simulink subsystem "control_initializer"  (R2023a)
settings: Solver=VariableStepAuto  StartTime=0.0  StopTime=10.0  RelTol=1e-3
libraries: sharedtransform x1
settings Model: Creator=thesa  LastModifiedBy=thesa

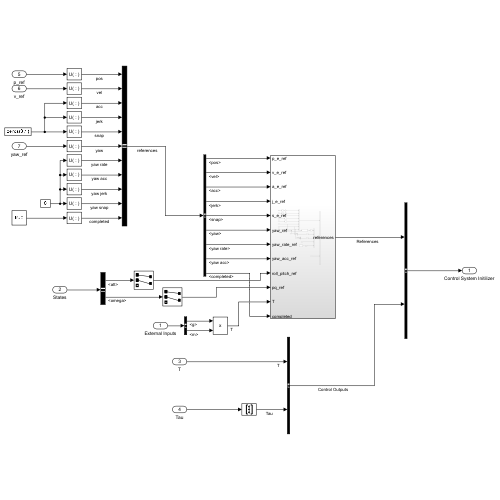
[thumbnail: Simulink's stored preview of the top-level diagram]
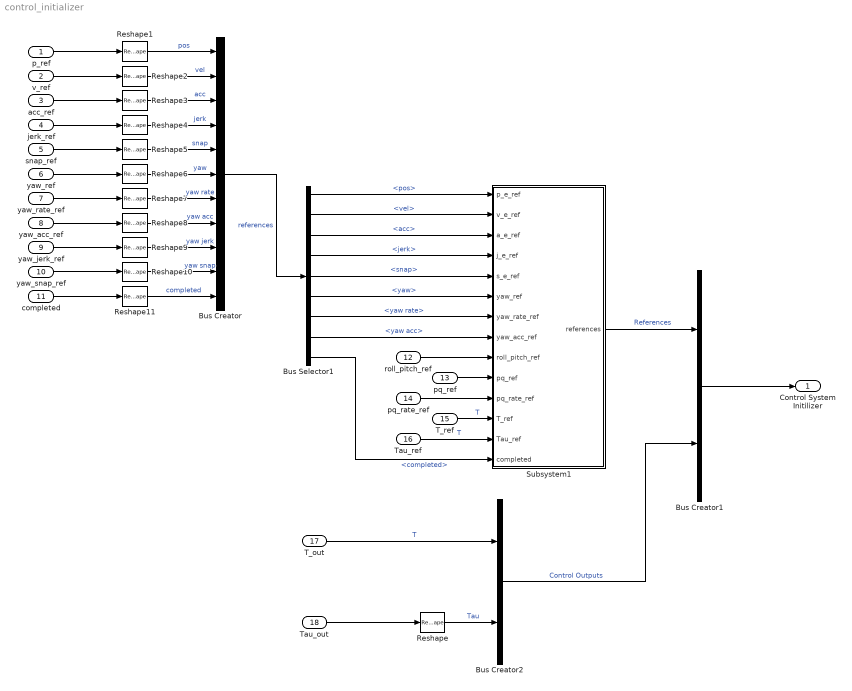
== system control_initializer ==
  p_ref : Inport
  v_ref : Inport  Port=2
  acc_ref : Inport  Port=3
  jerk_ref : Inport  Port=4
  snap_ref : Inport  Port=5
  yaw_ref : Inport  Port=6
  yaw_rate_ref : Inport  Port=7
  yaw_acc_ref : Inport  Port=8
  yaw_jerk_ref : Inport  Port=9
  yaw_snap_ref : Inport  Port=10
  completed : Inport  Port=11
  roll_pitch_ref : Inport  Port=12
  pq_ref : Inport  Port=13
  pq_rate_ref : Inport  Port=14
  T_ref : Inport  Port=15
  Tau_ref : Inport  Port=16
  T_out : Inport  Port=17
  Tau_out : Inport  Port=18
  Bus Creator : BusCreator  Inputs=11
  Bus Creator1 : BusCreator  Inputs=2
  Bus Creator2 : BusCreator  Inputs=2
  Bus Selector1 : BusSelector  OutputSignals=pos,vel,acc,jerk,snap,yaw,yaw rate,yaw acc,completed
  Reshape : Reshape  OutputDimensionality=Column vector (2-D)
  Reshape{1..11} (11 alike) : Reshape
  Subsystem1 : Subsystem
  Control System Initilizer : Outport
  wires:
  Reshape9/1 -> Bus Creator/9  "yaw jerk"
  Reshape5/1 -> Bus Creator/5  "snap"
  Reshape2/1 -> Bus Creator/2  "vel"
  Reshape6/1 -> Bus Creator/6  "yaw"
  T_out/1 -> Bus Creator2/1  "T"
  Bus Selector1/7 -> Subsystem1/7(yaw_rate_ref)  "<yaw rate>"
  Reshape11/1 -> Bus Creator/11  "completed"
  Reshape8/1 -> Bus Creator/8  "yaw acc"
  Reshape10/1 -> Bus Creator/10  "yaw snap"
  Subsystem1/1(references) -> Bus Creator1/1  "References"
  Bus Selector1/2 -> Subsystem1/2(v_e_ref)  "<vel>"
  Bus Selector1/4 -> Subsystem1/4(j_e_ref)  "<jerk>"
  p_ref/1 -> Reshape1/1
  Reshape1/1 -> Bus Creator/1  "pos"
  Bus Selector1/5 -> Subsystem1/5(s_e_ref)  "<snap>"
  Bus Creator1/1 -> Control System Initilizer/1
  Bus Selector1/9 -> Subsystem1/14(completed)  "<completed>"
  Reshape7/1 -> Bus Creator/7  "yaw rate"
  Bus Selector1/6 -> Subsystem1/6(yaw_ref)  "<yaw>"
  Bus Creator/1 -> Bus Selector1/1  "references"
  Bus Creator2/1 -> Bus Creator1/2  "Control Outputs"
  T_ref/1 -> Subsystem1/12(T_ref)  "T"
  Bus Selector1/1 -> Subsystem1/1(p_e_ref)  "<pos>"
  Reshape4/1 -> Bus Creator/4  "jerk"
  v_ref/1 -> Reshape2/1
  Bus Selector1/3 -> Subsystem1/3(a_e_ref)  "<acc>"
  yaw_ref/1 -> Reshape6/1
  Bus Selector1/8 -> Subsystem1/8(yaw_acc_ref)  "<yaw acc>"
  Reshape/1 -> Bus Creator2/2  "Tau"
  Tau_out/1 -> Reshape/1
  Reshape3/1 -> Bus Creator/3  "acc"
  jerk_ref/1 -> Reshape4/1
  acc_ref/1 -> Reshape3/1
  snap_ref/1 -> Reshape5/1
  yaw_rate_ref/1 -> Reshape7/1
  yaw_acc_ref/1 -> Reshape8/1
  yaw_jerk_ref/1 -> Reshape9/1
  yaw_snap_ref/1 -> Reshape10/1
  completed/1 -> Reshape11/1
  roll_pitch_ref/1 -> Subsystem1/9(roll_pitch_ref)
  Tau_ref/1 -> Subsystem1/13(Tau_ref)  "T"
  pq_rate_ref/1 -> Subsystem1/11(pq_rate_ref)
  pq_ref/1 -> Subsystem1/10(pq_ref)

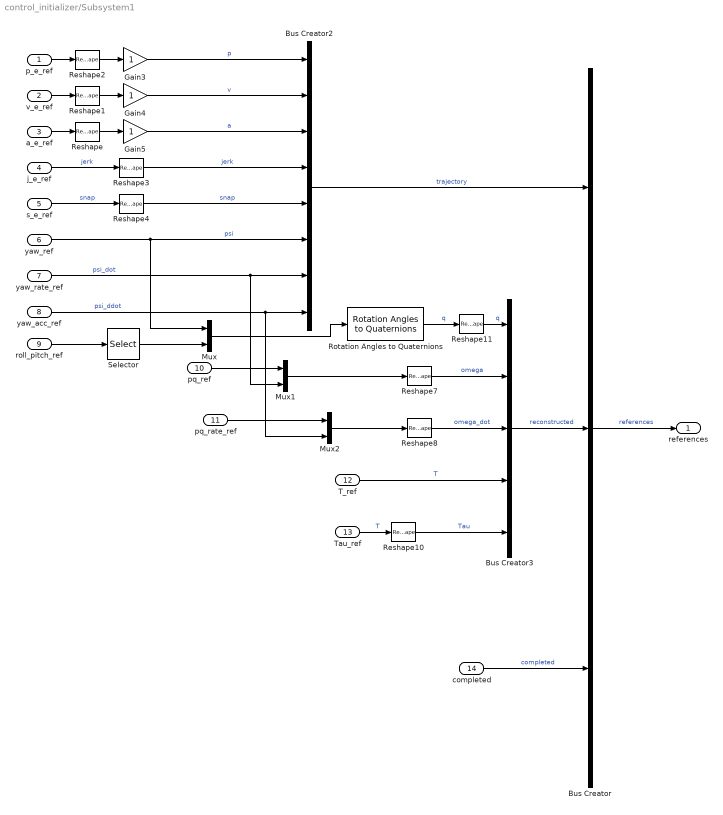
== system control_initializer/Subsystem1 ==
  p_e_ref : Inport
  v_e_ref : Inport  Port=2
  a_e_ref : Inport  Port=3
  j_e_ref : Inport  Port=4
  s_e_ref : Inport  Port=5
  yaw_ref : Inport  Port=6
  yaw_rate_ref : Inport  Port=7
  yaw_acc_ref : Inport  Port=8
  roll_pitch_ref : Inport  Port=9
  pq_ref : Inport  Port=10
  pq_rate_ref : Inport  Port=11
  T_ref : Inport  Port=12
  Tau_ref : Inport  Port=13
  completed : Inport  Port=14
  Bus Creator : BusCreator  Inputs=3
  Bus Creator2 : BusCreator  Inputs=8
  Bus Creator3 : BusCreator  Inputs=5
  Gain3 : Gain
  Gain4 : Gain
  Gain5 : Gain
  Mux : Mux  Inputs=2
  Mux1 : Mux  Inputs=2
  Mux2 : Mux  Inputs=2
  Reshape{,1..4,7..8,10} (8 alike) : Reshape  OutputDimensionality=Column vector (2-D)
  Reshape11 : Reshape  OutputDimensionality=Row vector (2-D)
  Rotation Angles to Quaternions : sharedtransform/Rotation Angles to Quaternions  rotationOrder=ZYX  aMode=aMode
  Selector : Selector  InputPortWidth=2  IndexOptions=Index vector (dialog)  Indices=[2 1]  OutputSizes=1
  references : Outport
  wires:
  pq_rate_ref/1 -> Mux2/1
  Tau_ref/1 -> Reshape10/1  "T"
  Reshape4/1 -> Bus Creator2/5  "snap"
  Reshape3/1 -> Bus Creator2/4  "jerk"
  Reshape2/1 -> Gain3/1
  Reshape1/1 -> Gain4/1
  Reshape/1 -> Gain5/1
  p_e_ref/1 -> Reshape2/1
  Gain3/1 -> Bus Creator2/1  "p"
  Gain5/1 -> Bus Creator2/3  "a"
  j_e_ref/1 -> Reshape3/1  "jerk"
  s_e_ref/1 -> Reshape4/1  "snap"
  yaw_ref/1 -> Bus Creator2/6, Mux/1  "psi"
  Gain4/1 -> Bus Creator2/2  "v"
  yaw_rate_ref/1 -> Mux1/2, Bus Creator2/7  "psi_dot"
  yaw_acc_ref/1 -> Bus Creator2/8, Mux2/2  "psi_ddot"
  pq_ref/1 -> Mux1/1
  Bus Creator/1 -> references/1  "references"
  T_ref/1 -> Bus Creator3/4  "T"
  Reshape7/1 -> Bus Creator3/2  "omega"
  Rotation Angles to Quaternions/1 -> Reshape11/1  "q"
  Reshape8/1 -> Bus Creator3/3  "omega_dot"
  Reshape11/1 -> Bus Creator3/1  "q"
  v_e_ref/1 -> Reshape1/1
  a_e_ref/1 -> Reshape/1
  Bus Creator3/1 -> Bus Creator/2  "reconstructed"
  Bus Creator2/1 -> Bus Creator/1  "trajectory"
  Mux2/1 -> Reshape8/1
  Reshape10/1 -> Bus Creator3/5  "Tau"
  Mux/1 -> Rotation Angles to Quaternions/1
  roll_pitch_ref/1 -> Selector/1
  Selector/1 -> Mux/2
  Mux1/1 -> Reshape7/1
  completed/1 -> Bus Creator/3  "completed"
